simulink model "split_factor_test"  (R2022a)
settings: Solver=VariableStepAuto  StartTime=0.0  StopTime=10.0  RelTol=1e-3
settings Model: Creator=Mick  LastModifiedBy=Mick

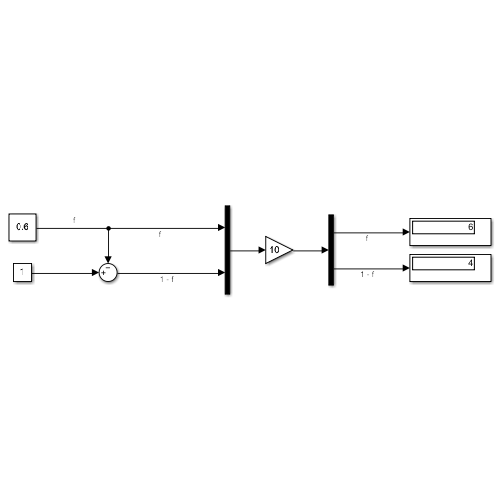
[thumbnail: Simulink's stored preview of the top-level diagram]
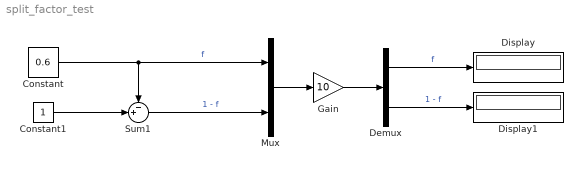
== system split_factor_test ==
  Constant : Constant  Value=0.6
  Constant1 : Constant
  Demux : Demux  Outputs=2
  Display : Display
  Display1 : Display
  Gain : Gain  Gain=10
  Mux : Mux  Inputs=2
  Sum1 : Sum  Inputs=-+|
  wires:
  Gain/1 -> Demux/1
  Mux/1 -> Gain/1
  Sum1/1 -> Mux/2  "1 - f"
  Constant/1 -> Mux/1, Sum1/1  "f"
  Constant1/1 -> Sum1/2
  Demux/1 -> Display/1  "f"
  Demux/2 -> Display1/1  "1 - f"
